simulink model "test_mdl1"  (R2023a)
settings: Solver=VariableStepAuto  StartTime=0.0  StopTime=10.0  RelTol=1e-3
(part 8 of 8)

== system test_mdl1/VehicleCAN/SOBDMC_HPCM_FD1/Cluster_HEV_Data4_FD1 ==
  BattChrgCmpltPt_T_Est : Constant  Value=0
  BattChrgTrgSocPt_T_Est : Constant  Value=0
  BattChrgTrgtLPt_T_Est : Constant  Value=0
  BattElec%f_D_Actl : Constant  Value=0
  bus_creator : BusCreator  Inputs=4
  out_port : Outport
  wires:
  bus_creator/1 -> out_port/1  "test_mdl1"
  BattChrgCmpltPt_T_Est/1 -> bus_creator/1  "BattChrgCmpltPt_T_Est"
  BattChrgTrgSocPt_T_Est/1 -> bus_creator/2  "BattChrgTrgSocPt_T_Est"
  BattChrgTrgtLPt_T_Est/1 -> bus_creator/3  "BattChrgTrgtLPt_T_Est"
  BattElec%f_D_Actl/1 -> bus_creator/4  "BattElec%f_D_Actl"

== system test_mdl1/VehicleCAN/SOBDMC_HPCM_FD1/Cluster_HEV_Data5 ==
  HybMdeStat_D_Dsply : Constant  Value=0
  PlgActvArb_B_Dsply : Constant  Value=0
  bus_creator : BusCreator  Inputs=2
  out_port : Outport
  wires:
  bus_creator/1 -> out_port/1  "test_mdl1"
  HybMdeStat_D_Dsply/1 -> bus_creator/1  "HybMdeStat_D_Dsply"
  PlgActvArb_B_Dsply/1 -> bus_creator/2  "PlgActvArb_B_Dsply"

== system test_mdl1/VehicleCAN/SOBDMC_HPCM_FD1/Cluster_HEV_Data7_FD1 ==
  BrkEvntComplt_B_Dsply : Constant  Value=0
  PreCondStat_D_Dsply : Constant  Value=0
  RgenEvntLvl_Pc_Dsply : Constant  Value=0
  bus_creator : BusCreator  Inputs=3
  out_port : Outport
  wires:
  bus_creator/1 -> out_port/1  "test_mdl1"
  BrkEvntComplt_B_Dsply/1 -> bus_creator/1  "BrkEvntComplt_B_Dsply"
  PreCondStat_D_Dsply/1 -> bus_creator/2  "PreCondStat_D_Dsply"
  RgenEvntLvl_Pc_Dsply/1 -> bus_creator/3  "RgenEvntLvl_Pc_Dsply"

== system test_mdl1/VehicleCAN/SOBDMC_HPCM_FD1/Cluster_HEV_Data9_FD1 ==
  MtrTrac2_Tq_Actl : Constant  Value=0
  NtfctnConflict1_D_Rq : Constant  Value=0
  OfbChrgSetSync_D_Stat : Constant  Value=0
  PtRmtRprt_D_Rq : Constant  Value=0
  bus_creator : BusCreator  Inputs=4
  out_port : Outport
  wires:
  bus_creator/1 -> out_port/1  "test_mdl1"
  MtrTrac2_Tq_Actl/1 -> bus_creator/1  "MtrTrac2_Tq_Actl"
  NtfctnConflict1_D_Rq/1 -> bus_creator/2  "NtfctnConflict1_D_Rq"
  OfbChrgSetSync_D_Stat/1 -> bus_creator/3  "OfbChrgSetSync_D_Stat"
  PtRmtRprt_D_Rq/1 -> bus_creator/4  "PtRmtRprt_D_Rq"

== system test_mdl1/VehicleCAN/SOBDMC_HPCM_FD1/ConsTip_Data_FD1 ==
  ConsTipV_No_Dsply : Constant  Value=0
  bus_creator : BusCreator  Inputs=1
  out_port : Outport
  wires:
  bus_creator/1 -> out_port/1  "test_mdl1"
  ConsTipV_No_Dsply/1 -> bus_creator/1  "ConsTipV_No_Dsply"

== system test_mdl1/VehicleCAN/SOBDMC_HPCM_FD1/GWM_HPCM_i_FrP10_FD1 ==
  ActChrgEndDay_No_Actl : Constant  Value=0
  ActChrgEndHr_No_Actl : Constant  Value=0
  ActChrgEndMin_No_Actl : Constant  Value=0
  ActChrgEndMnth_No_Actl : Constant  Value=0
  ActChrgEndYr_No2_Actl : Constant  Value=0
  ActChrgEndYr_No_Actl : Constant  Value=0
  BattChrgTrgtLMin_T_Est : Constant  Value=0
  bus_creator : BusCreator  Inputs=7
  out_port : Outport
  wires:
  bus_creator/1 -> out_port/1  "test_mdl1"
  ActChrgEndDay_No_Actl/1 -> bus_creator/1  "ActChrgEndDay_No_Actl"
  ActChrgEndHr_No_Actl/1 -> bus_creator/2  "ActChrgEndHr_No_Actl"
  ActChrgEndMin_No_Actl/1 -> bus_creator/3  "ActChrgEndMin_No_Actl"
  ActChrgEndMnth_No_Actl/1 -> bus_creator/4  "ActChrgEndMnth_No_Actl"
  ActChrgEndYr_No2_Actl/1 -> bus_creator/5  "ActChrgEndYr_No2_Actl"
  ActChrgEndYr_No_Actl/1 -> bus_creator/6  "ActChrgEndYr_No_Actl"
  BattChrgTrgtLMin_T_Est/1 -> bus_creator/7  "BattChrgTrgtLMin_T_Est"

== system test_mdl1/VehicleCAN/SOBDMC_HPCM_FD1/GWM_HPCM_i_FrP11_FD1 ==
  ActChrgStrMnth_No_Actl : Constant  Value=0
  ActChrgStrtDay_No_Actl : Constant  Value=0
  ActChrgStrtHr_No_Actl : Constant  Value=0
  ActChrgStrtMin_No_Actl : Constant  Value=0
  ActChrgStrtYr_No2_Actl : Constant  Value=0
  ActChrgStrtYr_No_Actl : Constant  Value=0
  BattChrgTrgtLMax_T_Est : Constant  Value=0
  bus_creator : BusCreator  Inputs=7
  out_port : Outport
  wires:
  bus_creator/1 -> out_port/1  "test_mdl1"
  ActChrgStrMnth_No_Actl/1 -> bus_creator/1  "ActChrgStrMnth_No_Actl"
  ActChrgStrtDay_No_Actl/1 -> bus_creator/2  "ActChrgStrtDay_No_Actl"
  ActChrgStrtHr_No_Actl/1 -> bus_creator/3  "ActChrgStrtHr_No_Actl"
  ActChrgStrtMin_No_Actl/1 -> bus_creator/4  "ActChrgStrtMin_No_Actl"
  ActChrgStrtYr_No2_Actl/1 -> bus_creator/5  "ActChrgStrtYr_No2_Actl"
  ActChrgStrtYr_No_Actl/1 -> bus_creator/6  "ActChrgStrtYr_No_Actl"
  BattChrgTrgtLMax_T_Est/1 -> bus_creator/7  "BattChrgTrgtLMax_T_Est"

== system test_mdl1/VehicleCAN/SOBDMC_HPCM_FD1/Global_PATS_Target2_FD1 ==
  bus_creator : BusCreator  Inputs=3
  immoTarget2Cmd : Constant  Value=0
  immoTarget2Data : Constant  Value=0
  immoTarget2Status : Constant  Value=0
  out_port : Outport
  wires:
  bus_creator/1 -> out_port/1  "test_mdl1"
  immoTarget2Cmd/1 -> bus_creator/1  "immoTarget2Cmd"
  immoTarget2Data/1 -> bus_creator/2  "immoTarget2Data"
  immoTarget2Status/1 -> bus_creator/3  "immoTarget2Status"

== system test_mdl1/VehicleCAN/SOBDMC_HPCM_FD1/GoTimeSettings_FD1 ==
  ChrgGoTAllOn_B_Stat : Constant  Value=0
  ChrgGoTElement_B_Dsply : Constant  Value=0
  ChrgGoTElement_D_Stat : Constant  Value=0
  ChrgGoTExtHtrEnbl_B_Rq : Constant  Value=0
  ChrgGoTExtHtr_B_Stat : Constant  Value=0
  ChrgGoTHr_T_Stat : Constant  Value=0
  ChrgGoTMnte_D_Stat : Constant  Value=0
  ChrgGoTNext_D_Stat : Constant  Value=0
  ChrgGoTPrcond_D_Stat : Constant  Value=0
  ChrgGoTTouchEnbl_B_Rq : Constant  Value=0
  ChrgGoTTouch_B_Stat : Constant  Value=0
  ChrgLocIdCurnt_D_Uns : Constant  Value=0
  bus_creator : BusCreator  Inputs=12
  out_port : Outport
  wires:
  bus_creator/1 -> out_port/1  "test_mdl1"
  ChrgGoTAllOn_B_Stat/1 -> bus_creator/1  "ChrgGoTAllOn_B_Stat"
  ChrgGoTElement_B_Dsply/1 -> bus_creator/2  "ChrgGoTElement_B_Dsply"
  ChrgGoTElement_D_Stat/1 -> bus_creator/3  "ChrgGoTElement_D_Stat"
  ChrgGoTExtHtrEnbl_B_Rq/1 -> bus_creator/4  "ChrgGoTExtHtrEnbl_B_Rq"
  ChrgGoTExtHtr_B_Stat/1 -> bus_creator/5  "ChrgGoTExtHtr_B_Stat"
  ChrgGoTHr_T_Stat/1 -> bus_creator/6  "ChrgGoTHr_T_Stat"
  ChrgGoTMnte_D_Stat/1 -> bus_creator/7  "ChrgGoTMnte_D_Stat"
  ChrgGoTNext_D_Stat/1 -> bus_creator/8  "ChrgGoTNext_D_Stat"
  ChrgGoTPrcond_D_Stat/1 -> bus_creator/9  "ChrgGoTPrcond_D_Stat"
  ChrgGoTTouchEnbl_B_Rq/1 -> bus_creator/10  "ChrgGoTTouchEnbl_B_Rq"
  ChrgGoTTouch_B_Stat/1 -> bus_creator/11  "ChrgGoTTouch_B_Stat"
  ChrgLocIdCurnt_D_Uns/1 -> bus_creator/12  "ChrgLocIdCurnt_D_Uns"

== system test_mdl1/VehicleCAN/SOBDMC_HPCM_FD1/HEV_ChargeStat_FD1 ==
  ChargeNowDuration_St : Constant  Value=0
  EstmChrgTimeHP_St : Constant  Value=0
  EstmChrgTimeLP_St : Constant  Value=0
  NxtUsgSocEst_Pc_Dsply : Constant  Value=0
  VehElRngeNut_L_Dsply : Constant  Value=0
  bus_creator : BusCreator  Inputs=5
  out_port : Outport
  wires:
  bus_creator/1 -> out_port/1  "test_mdl1"
  ChargeNowDuration_St/1 -> bus_creator/1  "ChargeNowDuration_St"
  EstmChrgTimeHP_St/1 -> bus_creator/2  "EstmChrgTimeHP_St"
  EstmChrgTimeLP_St/1 -> bus_creator/3  "EstmChrgTimeLP_St"
  NxtUsgSocEst_Pc_Dsply/1 -> bus_creator/4  "NxtUsgSocEst_Pc_Dsply"
  VehElRngeNut_L_Dsply/1 -> bus_creator/5  "VehElRngeNut_L_Dsply"

== system test_mdl1/VehicleCAN/SOBDMC_HPCM_FD1/MHT_EV_Wakeup_FD1 ==
  BattChlrSov_B_Rq : Constant  Value=0
  BattChrgTrgtSoC_D_Rq : Constant  Value=0
  BattTracClntVlv_B_Rq : Constant  Value=0
  BattTracDrvSustn_B_Rq : Constant  Value=0
  BrkAppl_D_RqPt : Constant  Value=0
  CabinDrvSustn_B_Rq : Constant  Value=0
  CabnEvapSovFront_B_Rq : Constant  Value=0
  CabnEvapSovRear_B_Rq : Constant  Value=0
  ChrgNowEvnt_B_Stat : Constant  Value=0
  HeatCoreSovRear_B_Rq : Constant  Value=0
  HtrnClntFlw_D_Rq : Constant  Value=0
  HtrnCnnctPwr_B_Stat : Constant  Value=0
  HtrnDcdcDis_B_Rq : Constant  Value=0
  PreCondBatt_B_Actl : Constant  Value=0
  PtcHtr_D_Stat : Constant  Value=0
  WakeAlarm0_B_Typ : Constant  Value=0
  WakeAlarm0_T_Rq : Constant  Value=0
  bus_creator : BusCreator  Inputs=17
  out_port : Outport
  wires:
  bus_creator/1 -> out_port/1  "test_mdl1"
  BattChlrSov_B_Rq/1 -> bus_creator/1  "BattChlrSov_B_Rq"
  BattChrgTrgtSoC_D_Rq/1 -> bus_creator/2  "BattChrgTrgtSoC_D_Rq"
  BattTracClntVlv_B_Rq/1 -> bus_creator/3  "BattTracClntVlv_B_Rq"
  BattTracDrvSustn_B_Rq/1 -> bus_creator/4  "BattTracDrvSustn_B_Rq"
  BrkAppl_D_RqPt/1 -> bus_creator/5  "BrkAppl_D_RqPt"
  CabinDrvSustn_B_Rq/1 -> bus_creator/6  "CabinDrvSustn_B_Rq"
  CabnEvapSovFront_B_Rq/1 -> bus_creator/7  "CabnEvapSovFront_B_Rq"
  CabnEvapSovRear_B_Rq/1 -> bus_creator/8  "CabnEvapSovRear_B_Rq"
  ChrgNowEvnt_B_Stat/1 -> bus_creator/9  "ChrgNowEvnt_B_Stat"
  HeatCoreSovRear_B_Rq/1 -> bus_creator/10  "HeatCoreSovRear_B_Rq"
  HtrnClntFlw_D_Rq/1 -> bus_creator/11  "HtrnClntFlw_D_Rq"
  HtrnCnnctPwr_B_Stat/1 -> bus_creator/12  "HtrnCnnctPwr_B_Stat"
  HtrnDcdcDis_B_Rq/1 -> bus_creator/13  "HtrnDcdcDis_B_Rq"
  PreCondBatt_B_Actl/1 -> bus_creator/14  "PreCondBatt_B_Actl"
  PtcHtr_D_Stat/1 -> bus_creator/15  "PtcHtr_D_Stat"
  WakeAlarm0_B_Typ/1 -> bus_creator/16  "WakeAlarm0_B_Typ"
  WakeAlarm0_T_Rq/1 -> bus_creator/17  "WakeAlarm0_T_Rq"

== system test_mdl1/VehicleCAN/SOBDMC_HPCM_FD1/MtrTracData_1_FD1 ==
  Inv1_Te_Actl : Constant  Value=0
  Mtr2Aout_W_ActlMntr : Constant  Value=0
  Mtr2CntlTeAlrm_B_Stat : Constant  Value=0
  MtrTrac2Coil_Te_Actl : Constant  Value=0
  MtrTrac2Falt_B_Stat : Constant  Value=0
  MtrTrac2Inv_Te_Actl : Constant  Value=0
  MtrTrac2TeAlrm_B_Stat : Constant  Value=0
  MtrTrac2_I_Actl : Constant  Value=0
  MtrTrac2_U_Actl : Constant  Value=0
  bus_creator : BusCreator  Inputs=9
  out_port : Outport
  wires:
  bus_creator/1 -> out_port/1  "test_mdl1"
  Inv1_Te_Actl/1 -> bus_creator/1  "Inv1_Te_Actl"
  Mtr2Aout_W_ActlMntr/1 -> bus_creator/2  "Mtr2Aout_W_ActlMntr"
  Mtr2CntlTeAlrm_B_Stat/1 -> bus_creator/3  "Mtr2CntlTeAlrm_B_Stat"
  MtrTrac2Coil_Te_Actl/1 -> bus_creator/4  "MtrTrac2Coil_Te_Actl"
  MtrTrac2Falt_B_Stat/1 -> bus_creator/5  "MtrTrac2Falt_B_Stat"
  MtrTrac2Inv_Te_Actl/1 -> bus_creator/6  "MtrTrac2Inv_Te_Actl"
  MtrTrac2TeAlrm_B_Stat/1 -> bus_creator/7  "MtrTrac2TeAlrm_B_Stat"
  MtrTrac2_I_Actl/1 -> bus_creator/8  "MtrTrac2_I_Actl"
  MtrTrac2_U_Actl/1 -> bus_creator/9  "MtrTrac2_U_Actl"

== system test_mdl1/VehicleCAN/SOBDMC_HPCM_FD1/MtrTrac_Data2_FD1 ==
  ChrgStat_D_ActlMntr : Constant  Value=0
  HybVehMde_D_ActlMntr : Constant  Value=0
  Inv1Ain_I_ActlMntr : Constant  Value=0
  Mtr2State_D_ActlMntr : Constant  Value=0
  VehElRnge_L_Dsply : Constant  Value=0
  bus_creator : BusCreator  Inputs=5
  out_port : Outport
  wires:
  bus_creator/1 -> out_port/1  "test_mdl1"
  ChrgStat_D_ActlMntr/1 -> bus_creator/1  "ChrgStat_D_ActlMntr"
  HybVehMde_D_ActlMntr/1 -> bus_creator/2  "HybVehMde_D_ActlMntr"
  Inv1Ain_I_ActlMntr/1 -> bus_creator/3  "Inv1Ain_I_ActlMntr"
  Mtr2State_D_ActlMntr/1 -> bus_creator/4  "Mtr2State_D_ActlMntr"
  VehElRnge_L_Dsply/1 -> bus_creator/5  "VehElRnge_L_Dsply"

== system test_mdl1/VehicleCAN/SOBDMC_HPCM_FD1/OTAPhysSOBDMCtoGWM_FD1 ==
  OTAPhysHPCMtoGWM_ECG : Constant  Value=0
  bus_creator : BusCreator  Inputs=1
  out_port : Outport
  wires:
  bus_creator/1 -> out_port/1  "test_mdl1"
  OTAPhysHPCMtoGWM_ECG/1 -> bus_creator/1  "OTAPhysHPCMtoGWM_ECG"

== system test_mdl1/VehicleCAN/SOBDMC_HPCM_FD1/PARSEDHPCMtoGWM_ECG_FD1 ==
  PARSEDPhysHPCMtoGWM_ECG : Constant  Value=0
  bus_creator : BusCreator  Inputs=1
  out_port : Outport
  wires:
  bus_creator/1 -> out_port/1  "test_mdl1"
  PARSEDPhysHPCMtoGWM_ECG/1 -> bus_creator/1  "PARSEDPhysHPCMtoGWM_ECG"

== system test_mdl1/VehicleCAN/SOBDMC_HPCM_FD1/PARSEDPushSOBDMCtoGWM_FD1 ==
  PARSEDPhysHPCM2toGWM_ECG : Constant  Value=0
  bus_creator : BusCreator  Inputs=1
  out_port : Outport
  wires:
  bus_creator/1 -> out_port/1  "test_mdl1"
  PARSEDPhysHPCM2toGWM_ECG/1 -> bus_creator/1  "PARSEDPhysHPCM2toGWM_ECG"

== system test_mdl1/VehicleCAN/SOBDMC_HPCM_FD1/PreCond_Hev_Data1_FD1 ==
  BattChrgInhbt_D_Rq : Constant  Value=0
  ChrgStat_D2_Dsply : Constant  Value=0
  ChrgTMatch_B_Stat : Constant  Value=0
  HvacPrecondAC_D_Rq : Constant  Value=0
  HvacPrecondBlwr2_D_Rq : Constant  Value=0
  HvacPrecondMode2_D_Rq : Constant  Value=0
  HvacPrecondRecirc_D_Rq : Constant  Value=0
  HvacPrecond_Te_Rq : Constant  Value=0
  bus_creator : BusCreator  Inputs=8
  out_port : Outport
  wires:
  bus_creator/1 -> out_port/1  "test_mdl1"
  BattChrgInhbt_D_Rq/1 -> bus_creator/1  "BattChrgInhbt_D_Rq"
  ChrgStat_D2_Dsply/1 -> bus_creator/2  "ChrgStat_D2_Dsply"
  ChrgTMatch_B_Stat/1 -> bus_creator/3  "ChrgTMatch_B_Stat"
  HvacPrecondAC_D_Rq/1 -> bus_creator/4  "HvacPrecondAC_D_Rq"
  HvacPrecondBlwr2_D_Rq/1 -> bus_creator/5  "HvacPrecondBlwr2_D_Rq"
  HvacPrecondMode2_D_Rq/1 -> bus_creator/6  "HvacPrecondMode2_D_Rq"
  HvacPrecondRecirc_D_Rq/1 -> bus_creator/7  "HvacPrecondRecirc_D_Rq"
  HvacPrecond_Te_Rq/1 -> bus_creator/8  "HvacPrecond_Te_Rq"

== system test_mdl1/VehicleCAN/SOBDMC_HPCM_FD1/PreCond_Hev_Data2_FD1 ==
  BattTracClntFlw_Pc_Rq : Constant  Value=0
  BattTrac_I_EstVsc : Constant  Value=0
  DrvCondTpRrDefrs_B_Rq : Constant  Value=0
  HtrnAin_UHi_Actl : Constant  Value=0
  HtrnHvilOpen_B_Actl : Constant  Value=0
  HtrnMil_D_Rq : Constant  Value=0
  HtrnOvrTeLamp_B_Dsply : Constant  Value=0
  HtrnSrvcRqd_B_Dsply : Constant  Value=0
  PreCondActv_B_Actl : Constant  Value=0
  PtWakeupDeltaT_T_Rq : Constant  Value=0
  bus_creator : BusCreator  Inputs=10
  out_port : Outport
  wires:
  bus_creator/1 -> out_port/1  "test_mdl1"
  BattTracClntFlw_Pc_Rq/1 -> bus_creator/1  "BattTracClntFlw_Pc_Rq"
  BattTrac_I_EstVsc/1 -> bus_creator/2  "BattTrac_I_EstVsc"
  DrvCondTpRrDefrs_B_Rq/1 -> bus_creator/3  "DrvCondTpRrDefrs_B_Rq"
  HtrnAin_UHi_Actl/1 -> bus_creator/4  "HtrnAin_UHi_Actl"
  HtrnHvilOpen_B_Actl/1 -> bus_creator/5  "HtrnHvilOpen_B_Actl"
  HtrnMil_D_Rq/1 -> bus_creator/6  "HtrnMil_D_Rq"
  HtrnOvrTeLamp_B_Dsply/1 -> bus_creator/7  "HtrnOvrTeLamp_B_Dsply"
  HtrnSrvcRqd_B_Dsply/1 -> bus_creator/8  "HtrnSrvcRqd_B_Dsply"
  PreCondActv_B_Actl/1 -> bus_creator/9  "PreCondActv_B_Actl"
  PtWakeupDeltaT_T_Rq/1 -> bus_creator/10  "PtWakeupDeltaT_T_Rq"

== system test_mdl1/VehicleCAN/SOBDMC_HPCM_FD1/SOBDMC_AutoSar_NetMgmt_FD1 ==
  SOBDMC_AutoSarNMControl : Constant  Value=0
  SOBDMC_AutoSarNMNodeId : Constant  Value=0
  SOBDMC_AutoSarNMReserved{1..4} (4 alike) : Constant  Value=0
  SOBDMC_GWNMProxy : Constant  Value=0
  SOBDMC_GWOnBoardTester : Constant  Value=0
  bus_creator : BusCreator  Inputs=8
  out_port : Outport
  wires:
  bus_creator/1 -> out_port/1  "test_mdl1"
  SOBDMC_AutoSarNMControl/1 -> bus_creator/1  "SOBDMC_AutoSarNMControl"
  SOBDMC_AutoSarNMNodeId/1 -> bus_creator/2  "SOBDMC_AutoSarNMNodeId"
  SOBDMC_AutoSarNMReserved1/1 -> bus_creator/3  "SOBDMC_AutoSarNMReserved1"
  SOBDMC_AutoSarNMReserved2/1 -> bus_creator/4  "SOBDMC_AutoSarNMReserved2"
  SOBDMC_AutoSarNMReserved3/1 -> bus_creator/5  "SOBDMC_AutoSarNMReserved3"
  SOBDMC_AutoSarNMReserved4/1 -> bus_creator/6  "SOBDMC_AutoSarNMReserved4"
  SOBDMC_GWNMProxy/1 -> bus_creator/7  "SOBDMC_GWNMProxy"
  SOBDMC_GWOnBoardTester/1 -> bus_creator/8  "SOBDMC_GWOnBoardTester"

== system test_mdl1/VehicleCAN/SOBDMC_HPCM_FD1/SOBDMC_RapidData_Resp1_FD1 ==
  UUDTSOBDMCResponse1 : Constant  Value=0
  bus_creator : BusCreator  Inputs=1
  out_port : Outport
  wires:
  bus_creator/1 -> out_port/1  "test_mdl1"
  UUDTSOBDMCResponse1/1 -> bus_creator/1  "UUDTSOBDMCResponse1"

== system test_mdl1/VehicleCAN/SOBDMC_HPCM_FD1/SOBDMC_RapidData_Resp2_FD1 ==
  UUDTSOBDMCResponse2 : Constant  Value=0
  bus_creator : BusCreator  Inputs=1
  out_port : Outport
  wires:
  bus_creator/1 -> out_port/1  "test_mdl1"
  UUDTSOBDMCResponse2/1 -> bus_creator/1  "UUDTSOBDMCResponse2"

== system test_mdl1/VehicleCAN/SOBDMC_HPCM_FD1/SOBDMC_RapidData_Resp3_FD1 ==
  UUDTSOBDMCResponse3 : Constant  Value=0
  bus_creator : BusCreator  Inputs=1
  out_port : Outport
  wires:
  bus_creator/1 -> out_port/1  "test_mdl1"
  UUDTSOBDMCResponse3/1 -> bus_creator/1  "UUDTSOBDMCResponse3"

== system test_mdl1/VehicleCAN/SOBDMC_HPCM_FD1/SOBDMC_RapidData_Resp4_FD1 ==
  UUDTSOBDMCResponse4 : Constant  Value=0
  bus_creator : BusCreator  Inputs=1
  out_port : Outport
  wires:
  bus_creator/1 -> out_port/1  "test_mdl1"
  UUDTSOBDMCResponse4/1 -> bus_creator/1  "UUDTSOBDMCResponse4"

== system test_mdl1/VehicleCAN/SOBDMC_HPCM_FD1/Saved_Charge_Location_FD1 ==
  ChrgLocId_D_Sav : Constant  Value=0
  ChrgLocLattDeg_An_Sav : Constant  Value=0
  ChrgLocLattFrct_An_Sav : Constant  Value=0
  ChrgLocLattPostv_B_Sav : Constant  Value=0
  ChrgLocLongDeg_An_Sav : Constant  Value=0
  ChrgLocLongFrct_An_Sav : Constant  Value=0
  ChrgLocLongPostv_B_Sav : Constant  Value=0
  ChrgLocSaved_B_Dsply : Constant  Value=0
  ChrgNowCurnt_B_Dsply : Constant  Value=0
  bus_creator : BusCreator  Inputs=9
  out_port : Outport
  wires:
  bus_creator/1 -> out_port/1  "test_mdl1"
  ChrgLocId_D_Sav/1 -> bus_creator/1  "ChrgLocId_D_Sav"
  ChrgLocLattDeg_An_Sav/1 -> bus_creator/2  "ChrgLocLattDeg_An_Sav"
  ChrgLocLattFrct_An_Sav/1 -> bus_creator/3  "ChrgLocLattFrct_An_Sav"
  ChrgLocLattPostv_B_Sav/1 -> bus_creator/4  "ChrgLocLattPostv_B_Sav"
  ChrgLocLongDeg_An_Sav/1 -> bus_creator/5  "ChrgLocLongDeg_An_Sav"
  ChrgLocLongFrct_An_Sav/1 -> bus_creator/6  "ChrgLocLongFrct_An_Sav"
  ChrgLocLongPostv_B_Sav/1 -> bus_creator/7  "ChrgLocLongPostv_B_Sav"
  ChrgLocSaved_B_Dsply/1 -> bus_creator/8  "ChrgLocSaved_B_Dsply"
  ChrgNowCurnt_B_Dsply/1 -> bus_creator/9  "ChrgNowCurnt_B_Dsply"

== system test_mdl1/VehicleCAN/SOBDMC_HPCM_FD1/TesterPhysicalResSOBDMCFD1 ==
  TesterPhysicalResSOBDMC : Constant  Value=0
  bus_creator : BusCreator  Inputs=1
  out_port : Outport
  wires:
  bus_creator/1 -> out_port/1  "test_mdl1"
  TesterPhysicalResSOBDMC/1 -> bus_creator/1  "TesterPhysicalResSOBDMC"

== system test_mdl1/VehicleCAN/SOBDMC_HPCM_FD1/Unsaved_Charge_LocationFD1 ==
  ChrgLocId_D_Uns : Constant  Value=0
  ChrgLocLattDeg_An_Uns : Constant  Value=0
  ChrgLocLattFrct_An_Uns : Constant  Value=0
  ChrgLocLattPostv_B_Uns : Constant  Value=0
  ChrgLocLongDeg_An_Uns : Constant  Value=0
  ChrgLocLongFrct_An_Uns : Constant  Value=0
  ChrgLocLongPostv_B_Uns : Constant  Value=0
  bus_creator : BusCreator  Inputs=7
  out_port : Outport
  wires:
  bus_creator/1 -> out_port/1  "test_mdl1"
  ChrgLocId_D_Uns/1 -> bus_creator/1  "ChrgLocId_D_Uns"
  ChrgLocLattDeg_An_Uns/1 -> bus_creator/2  "ChrgLocLattDeg_An_Uns"
  ChrgLocLattFrct_An_Uns/1 -> bus_creator/3  "ChrgLocLattFrct_An_Uns"
  ChrgLocLattPostv_B_Uns/1 -> bus_creator/4  "ChrgLocLattPostv_B_Uns"
  ChrgLocLongDeg_An_Uns/1 -> bus_creator/5  "ChrgLocLongDeg_An_Uns"
  ChrgLocLongFrct_An_Uns/1 -> bus_creator/6  "ChrgLocLongFrct_An_Uns"
  ChrgLocLongPostv_B_Uns/1 -> bus_creator/7  "ChrgLocLongPostv_B_Uns"

== system test_mdl1/VehicleCAN/TCCM/AWD_Torque_Data ==
  PrplWhlTotTqRqMxAwd_No_Cnt : Constant  Value=0
  PrplWhlTotTqRqMxAwd_No_Cs : Constant  Value=0
  PrplWhlTot_Tq_RqMxAwd : Constant  Value=0
  bus_creator : BusCreator  Inputs=3
  out_port : Outport
  wires:
  bus_creator/1 -> out_port/1  "test_mdl1"
  PrplWhlTotTqRqMxAwd_No_Cnt/1 -> bus_creator/1  "PrplWhlTotTqRqMxAwd_No_Cnt"
  PrplWhlTotTqRqMxAwd_No_Cs/1 -> bus_creator/2  "PrplWhlTotTqRqMxAwd_No_Cs"
  PrplWhlTot_Tq_RqMxAwd/1 -> bus_creator/3  "PrplWhlTot_Tq_RqMxAwd"

== system test_mdl1/VehicleCAN/TCCM/Driveline_Data_1 ==
  Awd2wdLamp_D_RqDsply : Constant  Value=0
  AwdAutoLamp_D_RqDsply : Constant  Value=0
  AwdHiLamp_D_RqDsply : Constant  Value=0
  AwdLck_D_Stat : Constant  Value=0
  AwdLck_Tq_Rq : Constant  Value=0
  AwdLoLamp_D_RqDsply : Constant  Value=0
  AwdOffRoadMode_D_Stats : Constant  Value=0
  AwdRnge_D_Actl : Constant  Value=0
  AwdSrvcRqd_B_Rq : Constant  Value=0
  AwdStat_D_RqDsply : Constant  Value=0
  AwdSys_D_Stat : Constant  Value=0
  NtrlTowAvail_B_Stat : Constant  Value=0
  TrnAout_Tq_RqMx : Constant  Value=0
  bus_creator : BusCreator  Inputs=13
  out_port : Outport
  wires:
  bus_creator/1 -> out_port/1  "test_mdl1"
  Awd2wdLamp_D_RqDsply/1 -> bus_creator/1  "Awd2wdLamp_D_RqDsply"
  AwdAutoLamp_D_RqDsply/1 -> bus_creator/2  "AwdAutoLamp_D_RqDsply"
  AwdHiLamp_D_RqDsply/1 -> bus_creator/3  "AwdHiLamp_D_RqDsply"
  AwdLck_D_Stat/1 -> bus_creator/4  "AwdLck_D_Stat"
  AwdLck_Tq_Rq/1 -> bus_creator/5  "AwdLck_Tq_Rq"
  AwdLoLamp_D_RqDsply/1 -> bus_creator/6  "AwdLoLamp_D_RqDsply"
  AwdOffRoadMode_D_Stats/1 -> bus_creator/7  "AwdOffRoadMode_D_Stats"
  AwdRnge_D_Actl/1 -> bus_creator/8  "AwdRnge_D_Actl"
  AwdSrvcRqd_B_Rq/1 -> bus_creator/9  "AwdSrvcRqd_B_Rq"
  AwdStat_D_RqDsply/1 -> bus_creator/10  "AwdStat_D_RqDsply"
  AwdSys_D_Stat/1 -> bus_creator/11  "AwdSys_D_Stat"
  NtrlTowAvail_B_Stat/1 -> bus_creator/12  "NtrlTowAvail_B_Stat"
  TrnAout_Tq_RqMx/1 -> bus_creator/13  "TrnAout_Tq_RqMx"

== system test_mdl1/VehicleCAN/TCCM/Driveline_Data_2 ==
  LsdSrvcRqd_B_Rq : Constant  Value=0
  RearDiffFalt_D_Stat : Constant  Value=0
  RearDiffLckLamp_D_Rq : Constant  Value=0
  RearDiffLckMsg_D_Rq : Constant  Value=0
  RearDiffLck_Tq_Actl : Constant  Value=0
  SelDrvMdeAwd2_D_Stat : Constant  Value=0
  bus_creator : BusCreator  Inputs=6
  out_port : Outport
  wires:
  bus_creator/1 -> out_port/1  "test_mdl1"
  LsdSrvcRqd_B_Rq/1 -> bus_creator/1  "LsdSrvcRqd_B_Rq"
  RearDiffFalt_D_Stat/1 -> bus_creator/2  "RearDiffFalt_D_Stat"
  RearDiffLckLamp_D_Rq/1 -> bus_creator/3  "RearDiffLckLamp_D_Rq"
  RearDiffLckMsg_D_Rq/1 -> bus_creator/4  "RearDiffLckMsg_D_Rq"
  RearDiffLck_Tq_Actl/1 -> bus_creator/5  "RearDiffLck_Tq_Actl"
  SelDrvMdeAwd2_D_Stat/1 -> bus_creator/6  "SelDrvMdeAwd2_D_Stat"

== system test_mdl1/VehicleCAN/TCCM/TCCM_AutoSar_NetwkMgmt ==
  TCCM_AutoSarNMControl : Constant  Value=0
  TCCM_AutoSarNMNodeId : Constant  Value=0
  TCCM_AutoSarNMReserved{1..4} (4 alike) : Constant  Value=0
  TCCM_GWNMProxy : Constant  Value=0
  TCCM_GWOnBoardTester : Constant  Value=0
  bus_creator : BusCreator  Inputs=8
  out_port : Outport
  wires:
  bus_creator/1 -> out_port/1  "test_mdl1"
  TCCM_AutoSarNMControl/1 -> bus_creator/1  "TCCM_AutoSarNMControl"
  TCCM_AutoSarNMNodeId/1 -> bus_creator/2  "TCCM_AutoSarNMNodeId"
  TCCM_AutoSarNMReserved1/1 -> bus_creator/3  "TCCM_AutoSarNMReserved1"
  TCCM_AutoSarNMReserved2/1 -> bus_creator/4  "TCCM_AutoSarNMReserved2"
  TCCM_AutoSarNMReserved3/1 -> bus_creator/5  "TCCM_AutoSarNMReserved3"
  TCCM_AutoSarNMReserved4/1 -> bus_creator/6  "TCCM_AutoSarNMReserved4"
  TCCM_GWNMProxy/1 -> bus_creator/7  "TCCM_GWNMProxy"
  TCCM_GWOnBoardTester/1 -> bus_creator/8  "TCCM_GWOnBoardTester"

== system test_mdl1/VehicleCAN/TCCM/TesterPhysicalResTCCM ==
  TesterPhysicalResTCCM : Constant  Value=0
  bus_creator : BusCreator  Inputs=1
  out_port : Outport
  wires:
  bus_creator/1 -> out_port/1  "test_mdl1"
  TesterPhysicalResTCCM/1 -> bus_creator/1  "TesterPhysicalResTCCM"

== system test_mdl1/VehicleCAN/TCM_DSL/EngineData_1 ==
  SeatWorkSrfc_B_Falt : Constant  Value=0
  TrnIpcDsplyGear_D_Actl : Constant  Value=0
  TrnIpcDsplyGear_D_Stat : Constant  Value=0
  TrnIpcDsplyMde_D_Actl : Constant  Value=0
  TrnIpcDsplyMde_D_Stat : Constant  Value=0
  TrnIpcDsplyRng2_D_Actl : Constant  Value=0
  TrnIpcDsplyRng_D_Stat : Constant  Value=0
  bus_creator : BusCreator  Inputs=7
  out_port : Outport
  wires:
  bus_creator/1 -> out_port/1  "test_mdl1"
  SeatWorkSrfc_B_Falt/1 -> bus_creator/1  "SeatWorkSrfc_B_Falt"
  TrnIpcDsplyGear_D_Actl/1 -> bus_creator/2  "TrnIpcDsplyGear_D_Actl"
  TrnIpcDsplyGear_D_Stat/1 -> bus_creator/3  "TrnIpcDsplyGear_D_Stat"
  TrnIpcDsplyMde_D_Actl/1 -> bus_creator/4  "TrnIpcDsplyMde_D_Actl"
  TrnIpcDsplyMde_D_Stat/1 -> bus_creator/5  "TrnIpcDsplyMde_D_Stat"
  TrnIpcDsplyRng2_D_Actl/1 -> bus_creator/6  "TrnIpcDsplyRng2_D_Actl"
  TrnIpcDsplyRng_D_Stat/1 -> bus_creator/7  "TrnIpcDsplyRng_D_Stat"

== system test_mdl1/VehicleCAN/TCM_DSL/Gear_Shift_by_Wire_3 ==
  GearSelLck_D_Rq : Constant  Value=0
  PrkBrkActv_D_RqTrnGear : Constant  Value=0
  TrnCmdCnt_B_Actl : Constant  Value=0
  TrnCmdState_B_Actl : Constant  Value=0
  TrnDtpCmd_D_Actl : Constant  Value=0
  TrnGearCmd_No_Cnt : Constant  Value=0
  TrnGearCmd_No_Cs : Constant  Value=0
  TrnGearCmd_Pc_ActlPt : Constant  Value=0
  TrnGearMsgTxt_D_Rq : Constant  Value=0
  TrnGearNtmAllow_B_Stat : Constant  Value=0
  TrnGear_D_RqPt : Constant  Value=0
  TrnLvrV_D_Rq : Constant  Value=0
  TrnNtrlTowCmd_D_Actl : Constant  Value=0
  TrnSbwSysHlth_D_Actl : Constant  Value=0
  TrnValidGear_D_Cnfm : Constant  Value=0
  bus_creator : BusCreator  Inputs=15
  out_port : Outport
  wires:
  bus_creator/1 -> out_port/1  "test_mdl1"
  GearSelLck_D_Rq/1 -> bus_creator/1  "GearSelLck_D_Rq"
  PrkBrkActv_D_RqTrnGear/1 -> bus_creator/2  "PrkBrkActv_D_RqTrnGear"
  TrnCmdCnt_B_Actl/1 -> bus_creator/3  "TrnCmdCnt_B_Actl"
  TrnCmdState_B_Actl/1 -> bus_creator/4  "TrnCmdState_B_Actl"
  TrnDtpCmd_D_Actl/1 -> bus_creator/5  "TrnDtpCmd_D_Actl"
  TrnGearCmd_No_Cnt/1 -> bus_creator/6  "TrnGearCmd_No_Cnt"
  TrnGearCmd_No_Cs/1 -> bus_creator/7  "TrnGearCmd_No_Cs"
  TrnGearCmd_Pc_ActlPt/1 -> bus_creator/8  "TrnGearCmd_Pc_ActlPt"
  TrnGearMsgTxt_D_Rq/1 -> bus_creator/9  "TrnGearMsgTxt_D_Rq"
  TrnGearNtmAllow_B_Stat/1 -> bus_creator/10  "TrnGearNtmAllow_B_Stat"
  TrnGear_D_RqPt/1 -> bus_creator/11  "TrnGear_D_RqPt"
  TrnLvrV_D_Rq/1 -> bus_creator/12  "TrnLvrV_D_Rq"
  TrnNtrlTowCmd_D_Actl/1 -> bus_creator/13  "TrnNtrlTowCmd_D_Actl"
  TrnSbwSysHlth_D_Actl/1 -> bus_creator/14  "TrnSbwSysHlth_D_Actl"
  TrnValidGear_D_Cnfm/1 -> bus_creator/15  "TrnValidGear_D_Cnfm"

== system test_mdl1/VehicleCAN/TCM_DSL/PowertrainData_10 ==
  GearEngag_D_Actl : Constant  Value=0
  GearLvr_D_ActlDrv : Constant  Value=0
  GearPos_D_Actl : Constant  Value=0
  GearPos_D_Trg : Constant  Value=0
  GearPos_No_Cnt : Constant  Value=0
  GearPos_No_Cs : Constant  Value=0
  TrnIgnOffDly_T_Rq : Constant  Value=0
  TrnPrkSys_D_Actl : Constant  Value=0
  TrnRng_D_Rq : Constant  Value=0
  bus_creator : BusCreator  Inputs=9
  out_port : Outport
  wires:
  bus_creator/1 -> out_port/1  "test_mdl1"
  GearEngag_D_Actl/1 -> bus_creator/1  "GearEngag_D_Actl"
  GearLvr_D_ActlDrv/1 -> bus_creator/2  "GearLvr_D_ActlDrv"
  GearPos_D_Actl/1 -> bus_creator/3  "GearPos_D_Actl"
  GearPos_D_Trg/1 -> bus_creator/4  "GearPos_D_Trg"
  GearPos_No_Cnt/1 -> bus_creator/5  "GearPos_No_Cnt"
  GearPos_No_Cs/1 -> bus_creator/6  "GearPos_No_Cs"
  TrnIgnOffDly_T_Rq/1 -> bus_creator/7  "TrnIgnOffDly_T_Rq"
  TrnPrkSys_D_Actl/1 -> bus_creator/8  "TrnPrkSys_D_Actl"
  TrnRng_D_Rq/1 -> bus_creator/9  "TrnRng_D_Rq"

== system test_mdl1/VehicleCAN/TCM_DSL/TCM_AutoSar_NetworkMgt ==
  TCM_AutoSarNMControl : Constant  Value=0
  TCM_AutoSarNMNodeId : Constant  Value=0
  TCM_AutoSarNMReserved{1..4} (4 alike) : Constant  Value=0
  TCM_GWNMProxy : Constant  Value=0
  TCM_GWOnBoardTester : Constant  Value=0
  bus_creator : BusCreator  Inputs=8
  out_port : Outport
  wires:
  bus_creator/1 -> out_port/1  "test_mdl1"
  TCM_AutoSarNMControl/1 -> bus_creator/1  "TCM_AutoSarNMControl"
  TCM_AutoSarNMNodeId/1 -> bus_creator/2  "TCM_AutoSarNMNodeId"
  TCM_AutoSarNMReserved1/1 -> bus_creator/3  "TCM_AutoSarNMReserved1"
  TCM_AutoSarNMReserved2/1 -> bus_creator/4  "TCM_AutoSarNMReserved2"
  TCM_AutoSarNMReserved3/1 -> bus_creator/5  "TCM_AutoSarNMReserved3"
  TCM_AutoSarNMReserved4/1 -> bus_creator/6  "TCM_AutoSarNMReserved4"
  TCM_GWNMProxy/1 -> bus_creator/7  "TCM_GWNMProxy"
  TCM_GWOnBoardTester/1 -> bus_creator/8  "TCM_GWOnBoardTester"

== system test_mdl1/VehicleCAN/TCM_DSL/TCM_Rapid_Data_Response_1 ==
  UUDTTCMResponse1 : Constant  Value=0
  bus_creator : BusCreator  Inputs=1
  out_port : Outport
  wires:
  bus_creator/1 -> out_port/1  "test_mdl1"
  UUDTTCMResponse1/1 -> bus_creator/1  "UUDTTCMResponse1"

== system test_mdl1/VehicleCAN/TCM_DSL/TCM_Rapid_Data_Response_2 ==
  UUDTTCMResponse2 : Constant  Value=0
  bus_creator : BusCreator  Inputs=1
  out_port : Outport
  wires:
  bus_creator/1 -> out_port/1  "test_mdl1"
  UUDTTCMResponse2/1 -> bus_creator/1  "UUDTTCMResponse2"

== system test_mdl1/VehicleCAN/TCM_DSL/TesterPhysicalResTCM ==
  TesterPhysicalResTCM : Constant  Value=0
  bus_creator : BusCreator  Inputs=1
  out_port : Outport
  wires:
  bus_creator/1 -> out_port/1  "test_mdl1"
  TesterPhysicalResTCM/1 -> bus_creator/1  "TesterPhysicalResTCM"

== system test_mdl1/VehicleCAN/TCM_DSL/TransData_3 ==
  TrnAout_W_ActlUnfilt : Constant  Value=0
  bus_creator : BusCreator  Inputs=1
  out_port : Outport
  wires:
  bus_creator/1 -> out_port/1  "test_mdl1"
  TrnAout_W_ActlUnfilt/1 -> bus_creator/1  "TrnAout_W_ActlUnfilt"

== system test_mdl1/VehicleCAN/TCM_DSL/TransGearData ==
  GboxOil_Te_Actl : Constant  Value=0
  GearLvrPos_D_Actl : Constant  Value=0
  SelDrvMdeSwtch_D_Stat3 : Constant  Value=0
  TrnShifActv_B_Actl : Constant  Value=0
  TrnSrvcRqd_B_Rq : Constant  Value=0
  bus_creator : BusCreator  Inputs=5
  out_port : Outport
  wires:
  bus_creator/1 -> out_port/1  "test_mdl1"
  GboxOil_Te_Actl/1 -> bus_creator/1  "GboxOil_Te_Actl"
  GearLvrPos_D_Actl/1 -> bus_creator/2  "GearLvrPos_D_Actl"
  SelDrvMdeSwtch_D_Stat3/1 -> bus_creator/3  "SelDrvMdeSwtch_D_Stat3"
  TrnShifActv_B_Actl/1 -> bus_creator/4  "TrnShifActv_B_Actl"
  TrnSrvcRqd_B_Rq/1 -> bus_creator/5  "TrnSrvcRqd_B_Rq"

== system test_mdl1/VehicleCAN/TCM_DSL/TransGearData_2 ==
  TrnMsgTxt2_D_Rq : Constant  Value=0
  TrnMsgTxt_D_Rq : Constant  Value=0
  bus_creator : BusCreator  Inputs=2
  out_port : Outport
  wires:
  bus_creator/1 -> out_port/1  "test_mdl1"
  TrnMsgTxt2_D_Rq/1 -> bus_creator/1  "TrnMsgTxt2_D_Rq"
  TrnMsgTxt_D_Rq/1 -> bus_creator/2  "TrnMsgTxt_D_Rq"

== system test_mdl1/VehicleCAN/TSTR/TesterFunctionalReq_FD1 ==
  TesterFunctionalReq : Constant  Value=0
  bus_creator : BusCreator  Inputs=1
  out_port : Outport
  wires:
  bus_creator/1 -> out_port/1  "test_mdl1"
  TesterFunctionalReq/1 -> bus_creator/1  "TesterFunctionalReq"

== system test_mdl1/VehicleCAN/TSTR/TesterPhysicalReqABS ==
  TesterPhysicalReqABS : Constant  Value=0
  bus_creator : BusCreator  Inputs=1
  out_port : Outport
  wires:
  bus_creator/1 -> out_port/1  "test_mdl1"
  TesterPhysicalReqABS/1 -> bus_creator/1  "TesterPhysicalReqABS"

== system test_mdl1/VehicleCAN/TSTR/TesterPhysicalReqCCM ==
  TesterPhysicalReqCCM : Constant  Value=0
  bus_creator : BusCreator  Inputs=1
  out_port : Outport
  wires:
  bus_creator/1 -> out_port/1  "test_mdl1"
  TesterPhysicalReqCCM/1 -> bus_creator/1  "TesterPhysicalReqCCM"

== system test_mdl1/VehicleCAN/TSTR/TesterPhysicalReqCMR_DSMC ==
  TesterPhysicalReqCMR_DSMC : Constant  Value=0
  bus_creator : BusCreator  Inputs=1
  out_port : Outport
  wires:
  bus_creator/1 -> out_port/1  "test_mdl1"
  TesterPhysicalReqCMR_DSMC/1 -> bus_creator/1  "TesterPhysicalReqCMR_DSMC"

== system test_mdl1/VehicleCAN/TSTR/TesterPhysicalReqGWM_FD1 ==
  TesterPhysicalReqGWM_F1 : Constant  Value=0
  bus_creator : BusCreator  Inputs=1
  out_port : Outport
  wires:
  bus_creator/1 -> out_port/1  "test_mdl1"
  TesterPhysicalReqGWM_F1/1 -> bus_creator/1  "TesterPhysicalReqGWM_F1"

== system test_mdl1/VehicleCAN/TSTR/TesterPhysicalReqIPMA ==
  TesterPhysicalReqIPMA : Constant  Value=0
  bus_creator : BusCreator  Inputs=1
  out_port : Outport
  wires:
  bus_creator/1 -> out_port/1  "test_mdl1"
  TesterPhysicalReqIPMA/1 -> bus_creator/1  "TesterPhysicalReqIPMA"

== system test_mdl1/VehicleCAN/TSTR/TesterPhysicalReqPCM ==
  TesterPhysicalReqPCM : Constant  Value=0
  bus_creator : BusCreator  Inputs=1
  out_port : Outport
  wires:
  bus_creator/1 -> out_port/1  "test_mdl1"
  TesterPhysicalReqPCM/1 -> bus_creator/1  "TesterPhysicalReqPCM"

== system test_mdl1/VehicleCAN/TSTR/TesterPhysicalReqPSCM ==
  TesterPhysicalReqPSCM : Constant  Value=0
  bus_creator : BusCreator  Inputs=1
  out_port : Outport
  wires:
  bus_creator/1 -> out_port/1  "test_mdl1"
  TesterPhysicalReqPSCM/1 -> bus_creator/1  "TesterPhysicalReqPSCM"

== system test_mdl1/VehicleCAN/TSTR/TesterPhysicalReqSOBDMC_FD ==
  TesterPhysicalReqSOBDMC : Constant  Value=0
  bus_creator : BusCreator  Inputs=1
  out_port : Outport
  wires:
  bus_creator/1 -> out_port/1  "test_mdl1"
  TesterPhysicalReqSOBDMC/1 -> bus_creator/1  "TesterPhysicalReqSOBDMC"

== system test_mdl1/VehicleCAN/TSTR/TesterPhysicalReqSODCMC ==
  TesterPhysicalReqSODCMC : Constant  Value=0
  bus_creator : BusCreator  Inputs=1
  out_port : Outport
  wires:
  bus_creator/1 -> out_port/1  "test_mdl1"
  TesterPhysicalReqSODCMC/1 -> bus_creator/1  "TesterPhysicalReqSODCMC"

== system test_mdl1/VehicleCAN/TSTR/TesterPhysicalReqSODCMD ==
  TesterPhysicalReqSODCMD : Constant  Value=0
  bus_creator : BusCreator  Inputs=1
  out_port : Outport
  wires:
  bus_creator/1 -> out_port/1  "test_mdl1"
  TesterPhysicalReqSODCMD/1 -> bus_creator/1  "TesterPhysicalReqSODCMD"

== system test_mdl1/VehicleCAN/TSTR/TesterPhysicalReqSODL ==
  TesterPhysicalReqSODL : Constant  Value=0
  bus_creator : BusCreator  Inputs=1
  out_port : Outport
  wires:
  bus_creator/1 -> out_port/1  "test_mdl1"
  TesterPhysicalReqSODL/1 -> bus_creator/1  "TesterPhysicalReqSODL"

== system test_mdl1/VehicleCAN/TSTR/TesterPhysicalReqSODR ==
  TesterPhysicalReqSODR : Constant  Value=0
  bus_creator : BusCreator  Inputs=1
  out_port : Outport
  wires:
  bus_creator/1 -> out_port/1  "test_mdl1"
  TesterPhysicalReqSODR/1 -> bus_creator/1  "TesterPhysicalReqSODR"

== system test_mdl1/VehicleCAN/TSTR/TesterPhysicalReqTCCM ==
  TesterPhysicalReqTCCM : Constant  Value=0
  bus_creator : BusCreator  Inputs=1
  out_port : Outport
  wires:
  bus_creator/1 -> out_port/1  "test_mdl1"
  TesterPhysicalReqTCCM/1 -> bus_creator/1  "TesterPhysicalReqTCCM"

== system test_mdl1/VehicleCAN/TSTR/TesterPhysicalReqTCM ==
  TesterPhysicalReqTCM : Constant  Value=0
  bus_creator : BusCreator  Inputs=1
  out_port : Outport
  wires:
  bus_creator/1 -> out_port/1  "test_mdl1"
  TesterPhysicalReqTCM/1 -> bus_creator/1  "TesterPhysicalReqTCM"

== system test_mdl1/VehicleCAN/VDM/Suspension_Data ==
  SuspClkSync_No_Rq : Constant  Value=0
  SuspFrntRight_L_Actl : Constant  Value=0
  SuspFrnt_L_Actl : Constant  Value=0
  SuspFrnt_L_Prev : Constant  Value=0
  SuspRearRight_L_Actl : Constant  Value=0
  SuspRear_L_Actl : Constant  Value=0
  SuspRear_L_Prev : Constant  Value=0
  bus_creator : BusCreator  Inputs=7
  out_port : Outport
  wires:
  bus_creator/1 -> out_port/1  "test_mdl1"
  SuspClkSync_No_Rq/1 -> bus_creator/1  "SuspClkSync_No_Rq"
  SuspFrntRight_L_Actl/1 -> bus_creator/2  "SuspFrntRight_L_Actl"
  SuspFrnt_L_Actl/1 -> bus_creator/3  "SuspFrnt_L_Actl"
  SuspFrnt_L_Prev/1 -> bus_creator/4  "SuspFrnt_L_Prev"
  SuspRearRight_L_Actl/1 -> bus_creator/5  "SuspRearRight_L_Actl"
  SuspRear_L_Actl/1 -> bus_creator/6  "SuspRear_L_Actl"
  SuspRear_L_Prev/1 -> bus_creator/7  "SuspRear_L_Prev"

== system test_mdl1/VehicleCAN/VDM/TesterPhysicalResVDM ==
  TesterPhysicalResVDM : Constant  Value=0
  bus_creator : BusCreator  Inputs=1
  out_port : Outport
  wires:
  bus_creator/1 -> out_port/1  "test_mdl1"
  TesterPhysicalResVDM/1 -> bus_creator/1  "TesterPhysicalResVDM"

== system test_mdl1/VehicleCAN/VDM/VeyDynamics_Data ==
  AdptDrvMdeChassis_D_Rq : Constant  Value=0
  AdptDrvMdePt_D_Rq : Constant  Value=0
  CcdMsgTxt_D_RqDsply : Constant  Value=0
  Ccd_B_Falt : Constant  Value=0
  SelDrvMdeSusp_D_Stat : Constant  Value=0
  bus_creator : BusCreator  Inputs=5
  out_port : Outport
  wires:
  bus_creator/1 -> out_port/1  "test_mdl1"
  AdptDrvMdeChassis_D_Rq/1 -> bus_creator/1  "AdptDrvMdeChassis_D_Rq"
  AdptDrvMdePt_D_Rq/1 -> bus_creator/2  "AdptDrvMdePt_D_Rq"
  CcdMsgTxt_D_RqDsply/1 -> bus_creator/3  "CcdMsgTxt_D_RqDsply"
  Ccd_B_Falt/1 -> bus_creator/4  "Ccd_B_Falt"
  SelDrvMdeSusp_D_Stat/1 -> bus_creator/5  "SelDrvMdeSusp_D_Stat"
